simulink model "microNole_MPC2019b"  (R2019b)
settings: Solver=VariableStepAuto  StartTime=0.0  StopTime=50  RelTol=1e-3
values from neighbouring files (symbols this model uses):
  b1 = Theta6*Vx + Theta5*Rw*omegam/rg    [run_model_MPC.m]
  b2 = Theta3*L*Vx/2 + Rw*L*Theta4*omegam/(2*rg)    [run_model_MPC.m]
  d0 = 0.1    [run_model_MPC.m]
  desired_longitudinal_speed = 2    [run_model_MPC.m]
  double_lane_flag = 0    [Trajectory_generator.m]
  K1 = Theta1*k5/(Theta2*k2)    [run_model_MPC.m]
  K_mpc_clock = optimal_regulation_controller(A_lat_d2,B1_lat_d2,e0,Q,R,h)    [run_model_MPC.m]
  K_mpc_counterclock = optimal_regulation_controller(A_lat_d,B1_lat_d,e0,Q,R,h)    [run_model_MPC.m]
  Ki1 = 0.48    [run_model_MPC.m]
  Kp1 = 0.3    [run_model_MPC.m]
  L = 0.256    [run_model_MPC.m]
  omegam0 = 0.0    (= 0)    [run_model_MPC.m]
  p1 = polyfit(z,f(z),2)    [Trajectory_generator.m]
  rg = 9.49    [run_model_MPC.m]
  Rw = 0.024    [run_model_MPC.m]
  sat_pwm = 0.2    [run_model_MPC.m]
  sat_steering = pi/6    (= 0.523598775598)    [run_model_MPC.m]
  Theta1 = 4.53547683764    [Thetas.mat]
  Theta2 = 12985.1550616    [Thetas.mat]
  Theta3 = 191.174871818    [Thetas.mat]
  Theta4 = 85.0179707731    [Thetas.mat]
  Theta5 = 696.470803284    [Thetas.mat]
  Theta6 = 370.37037037    [Thetas.mat]
  Ts = 0.01    [run_model_MPC.m]
  V0 = [0.0; 0.0; 0.0]    [run_model_MPC.m]
  X0 = [0.0; 0.0; 0.0]    [run_model_MPC.m]
libraries: simulink x1
settings Model: OrderedModelArguments=off  Creator=zysgh  LastModifiedBy=Abelb
settings DebuggingCC: SFMachineParentedDataDiag=error

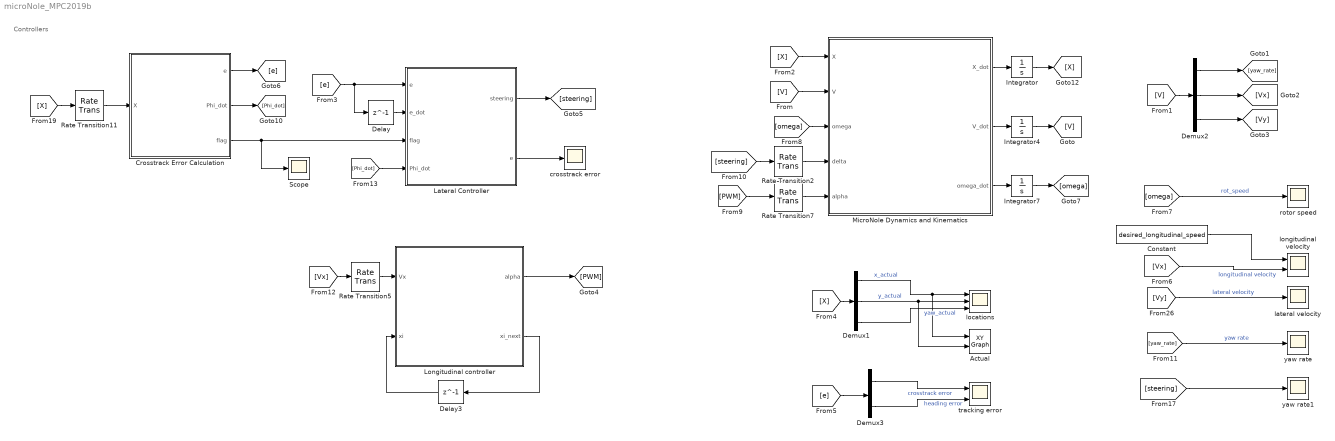
== system microNole_MPC2019b ==
  note: Controllers
  Actual : simulink/Sinks/XY Graph  xmin=0  xmax=50  ymin=-10  ymax=5  st=-1
  Constant : Constant  Value=desired_longitudinal_speed
  Crosstrack Error Calculation : MATLAB Function  TreatAsAtomicUnit=on
  Delay : Delay  DelayLength=1  InitialCondition=[e10; e20]  SampleTime=Ts
  Delay3 : Delay  DelayLength=1  SampleTime=Ts
  Demux1 : Demux  Outputs=3
  Demux2 : Demux  Outputs=3
  Demux3 : Demux  Outputs=2
  Integrator : Integrator  InitialCondition=X0
  Integrator4 : Integrator  InitialCondition=V0
  Integrator7 : Integrator  InitialCondition=omegam0
  Lateral Controller : MATLAB Function  TreatAsAtomicUnit=on
  Longitudinal controller : MATLAB Function  TreatAsAtomicUnit=on
  MicroNole Dynamics and Kinematics : MATLAB Function  TreatAsAtomicUnit=on
  Rate Transition11 : RateTransition  InitialCondition=X0  OutPortSampleTime=Ts
  Rate Transition2 : RateTransition  Integrity=off  OutPortSampleTime=0
  Rate Transition5 : RateTransition  OutPortSampleTime=Ts
  Rate Transition7 : RateTransition  Integrity=off  OutPortSampleTime=0
  Scope : Scope
  crosstrack error : Scope
  lateral velocity : Scope
  locations : Scope  NumInputPorts=3
  longitudinal velocity : Scope  NumInputPorts=2
  rotor speed : Scope
  tracking error : Scope  NumInputPorts=2
  yaw rate : Scope
  yaw rate1 : Scope
  wires:
  [X] -> Demux1/1
  Demux1/1 -> Actual/1, locations/1  "x_actual"
  Demux1/2 -> Actual/2, locations/2  "y_actual"
  Demux1/3 -> locations/3  "yaw_actual"
  MicroNole Dynamics and Kinematics/3(omega_dot) -> Integrator7/1
  [omega] -> rotor speed/1  "rot_speed"
  [Vy] -> lateral velocity/1  "lateral velocity"
  MicroNole Dynamics and Kinematics/2(V_dot) -> Integrator4/1
  [V] -> MicroNole Dynamics and Kinematics/2(V)
  [omega] -> MicroNole Dynamics and Kinematics/3(omega)
  Integrator7/1 -> [omega]
  Integrator4/1 -> [V]
  [V] -> Demux2/1
  Demux2/1 -> [yaw_rate]
  Demux2/2 -> [Vx]
  Demux2/3 -> [Vy]
  MicroNole Dynamics and Kinematics/1(X_dot) -> Integrator/1
  Integrator/1 -> [X]
  [X] -> MicroNole Dynamics and Kinematics/1(X)
  Delay3/1 -> Longitudinal controller/2(xi)
  [Vx] -> Rate Transition5/1
  Rate Transition5/1 -> Longitudinal controller/1(Vx)
  Longitudinal controller/2(xi_next) -> Delay3/1
  [X] -> Rate Transition11/1
  Lateral Controller/2(e) -> crosstrack error/1
  Lateral Controller/1(steering) -> [steering]
  Rate Transition11/1 -> Crosstrack Error Calculation/1(X)
  Crosstrack Error Calculation/1(e) -> [e]
  [Vx] -> longitudinal velocity/2  "longitudinal velocity"
  [yaw_rate] -> yaw rate/1  "yaw rate"
  [e] -> Demux3/1
  Demux3/1 -> tracking error/1  "crosstrack error"
  Demux3/2 -> tracking error/2  "heading error"
  Constant/1 -> longitudinal velocity/1
  [steering] -> Rate Transition2/1
  Rate Transition2/1 -> MicroNole Dynamics and Kinematics/4(delta)
  Longitudinal controller/1(alpha) -> [PWM]
  [PWM] -> Rate Transition7/1
  Rate Transition7/1 -> MicroNole Dynamics and Kinematics/5(alpha)
  Delay/1 -> Lateral Controller/2(e_dot)
  [e] -> Delay/1, Lateral Controller/1("e ")
  Crosstrack Error Calculation/2(Phi_dot) -> [Phi_dot]
  [Phi_dot] -> Lateral Controller/4(Phi_dot)
  [steering] -> yaw rate1/1
  Crosstrack Error Calculation/3(flag) -> Scope/1, Lateral Controller/3(flag)

== matlab function microNole_MPC2019b/MicroNole Dynamics and Kinematics ==
  data: X input; X_dot output; V input; V_dot output; omega input; delta input; alpha input; omega_dot output; Theta2 parameter; Theta3 parameter; Theta4 parameter; L parameter; Rw parameter; rg parameter; Theta1 parameter; Theta5 parameter; sat_pwm parameter; sat_steering parameter; d0 parameter
function [X_dot, V_dot, omega_dot] = fcn(X, V, omega, delta,alpha, Theta2, Theta3, Theta4, L, Rw, rg, Theta1, Theta5,sat_pwm, sat_steering,d0)
%%
% States:
%        - X: [x,y,heading] world frame
%        - V: [Vx, Vy, yaw rate] car frame
%        - yaw: car yaw angle
%        - omega: motor rotation speed
% Inputs: 
%        - delta: steering angle
%        - alpha: throttle command (PWM%)
% parameters:
%

% %% command satuation
% if abs(alpha) > sat_pwm
%     alpha =  sign(alpha) * sat_pwm;
% end
if abs(delta) > sat_steering
    delta =  sign(delta) * sat_steering;
end
%% upacking inputs
yaw_rate = V(1);
Vx = V(2);
Vy = V(3);
Phi = X(3);

%% dynamical model
Theta6 = Theta3*Theta5/Theta4;

omega_dot = -Theta1 * omega + Theta2 * alpha;

A1 = (L/2) * Theta3 * delta * cos(delta);
B1 = (L/2) * Theta3 *(1-cos(delta));
C1 = ((1/2) * Theta3 * (1+cos(delta)) + Theta4) * (1/2) * L^2;
D1 = (Rw*L/(2*rg)) * Theta4 * sin(delta);
yaw_rate_dot = -C1*yaw_rate + A1*Vx + B1*Vy + D1*omega;

A2 = 2 * Theta5 + Theta6 * delta * sin(delta);
B2 = Theta6 * sin(delta);
C2 = L*Theta6*sin(delta)/2;
D2 = Theta5*Rw*(1+cos(delta))/rg;
Vx_dot = -A2*Vx + B2*Vy + C2*yaw_rate + yaw_rate*Vy + D2*omega;

A3 = Theta6 * delta * cos(delta);
B3 = Theta6 * (1+cos(delta));
C3 = L*(Theta6*(1-cos(delta))-2*Theta5)/2;
D3 = Theta5 * Rw *sin(delta)/rg;
Vy_dot = -B3*Vy + A3*Vx + C3*yaw_rate - yaw_rate*Vx + D3*omega;

%% forward kinematics (bickycle)
v = sqrt(Vx^2 + Vy^2);
beta = atan(tan(delta)/2);

x_dot = v * cos(Phi + beta);
y_dot = v * sin(Phi + beta);
Phi_dot = v * cos(beta) * tan(delta) / L;
% Phi_dot = yaw_rate;

% %% crosstrack kinematics
% ePhi = Phi_ref - Phi;
% d_dot = d0 - ((L*yaw_rate/2) * cos(ePhi) - Vx * sin(ePhi));



%% packing outputs
V_dot = [yaw_rate_dot;
         Vx_dot;
         Vy_dot];
     
X_dot = [x_dot;
         y_dot;
         Phi_dot];

== matlab function microNole_MPC2019b/Longitudinal controller ==
  data: Vx input; xi input; Kp1 parameter; Ki1 parameter; K1 parameter; alpha output; xi_next output; Ts parameter; desired_longitudinal_speed parameter
function [alpha,xi_next] = fcn(Vx, xi, Kp1, Ki1,K1, Ts, desired_longitudinal_speed)
%% function [alpha,delta] = fcn(eVx, eOmegaz)
% low_level controller (PID) for yaw rate and longitudinal velocity
% Inputs:
%        - eVx: longitudinal velocity error = Vx_desired - Vx
%        - eOmegaz: yaw rate error = Omegaz_desired - Omegaz
% Outputs:
%        - alpha: PWM
%        - delta: steering angle
%
% Yu Zheng, RasLab, 01/04/2022

%% longitudinal velocity controller (PI)
eVx = desired_longitudinal_speed - Vx;
tau1 = 1;
tau2 = 1;
xi_next =  tau1 * xi + tau2 * eVx*Ts ;
alpha = K1 * desired_longitudinal_speed + Kp1 * eVx + Ki1 * xi;

== matlab function microNole_MPC2019b/Crosstrack Error Calculation ==
  data: X input; p1 parameter; e output; double_lane_flag parameter; Phi_dot output; flag output
function [e,Phi_dot,flag] = fcn(X,p1,double_lane_flag)
% for double trajectory: [e,Phi_dot,flag] = fcn(X,p1,p2, x_boundary,double_lane_flag)
% for single trajectory: [e,Phi_dot,flag] = fcn(X,p1,double_lane_flag)


%% crosstrack error calculation
x = X(1);
y = X(2);
omegaz = X(3);


% %%%%%%%%%%%% 2. polynomial  %%%%%%%%%%%%
p = p1;
if double_lane_flag == 1  % if there exists double trajectorys?
    if x <= x_boundary
        p = p1;
    else
        p = p2;
    end
end
[e1,e2,Phi_dot,flag] = crosstrack_error(x,y,p,omegaz);

e = [e1;
     e2];

== matlab function microNole_MPC2019b/Lateral Controller ==
  data: e input; e_dot input; K_mpc_clock parameter; b1 parameter; b2 parameter; flag input; Phi_dot input; Theta5 parameter; Theta6 parameter; Theta3 parameter; Theta4 parameter; L parameter; steering output; e output; desired_longitudinal_speed parameter; K_mpc_counterclock parameter
function [steering,e] = fcn(e, e_dot, K_mpc_clock,b1, b2,flag,Phi_dot, Theta5, Theta6, Theta3, Theta4, L,desired_longitudinal_speed, K_mpc_counterclock)

E = [e(1);e_dot(1);e(2);e_dot(2)];

%% controller
K_mpc = K_mpc_counterclock;
% 1: counter clockwise; -1: clockwise
if flag == -1
    K_mpc = K_mpc_clock;
end
    
% feedforward term
% the steady error on lateral distance could be vanished
% the steady error on heading error could not be vanished, it is because
% the slips angles at the rear and front wheels are completely determined.
Vx = desired_longitudinal_speed;
if Phi_dot == 0
    delta_ff = 0;
else
    R = Vx/Phi_dot;
    delta_ff = -K_mpc(3)*(Theta5-Vx)/(2*R*Theta6) + (L^2)*Vx*(Theta3+Theta4)/(2*R*b2) - b1*K_mpc(3)*(L^2)*(Theta3+Theta4)/(4*R*Theta6*b2);
end

% feeback
% steering = k_mpc * E + 2*sign(E)*d0;
steering = K_mpc * E + delta_ff;
